simulink model "controller_imp"  (R2024b)
settings: Solver=FixedStepDiscrete  StartTime=0.0  StopTime=1000  FixedStep=1/10  RelTol=1e-3  EnableMultiTasking=on
undefined symbols (not defined in the file): MAX_RDB_ENGAGE_SPEED, MAX_TORQUE, MAX_TORQUE_REVERSE, TransmissionState
libraries: arduinolib x18
settings Model: ExtModeTrigDuration=2  Creator=DAUIN-Win10  LastModifiedBy=feder
settings SolverCC: AutoInsertRateTranBlk=on
settings OptimizationCC: EnhancedBackFolding=on  PassReuseOutputArgsAs=Individual arguments  ZeroExternalMemoryAtStartup=off  ZeroInternalMemoryAtStartup=off  MaxStackSize=64  OptimizeBlockOrder=speed  DifferentSizesBufferReuse=on  OptimizationCustomize=off  EfficientTunableParamExpr=on
settings DebuggingCC: ParameterTunabilityLossMsg=error  UnconnectedInputMsg=warning  UnconnectedOutputMsg=warning  UnconnectedLineMsg=warning
settings HardwareCC: ProdBitPerInt=16  ProdBitPerPointer=16  ProdBitPerSizeT=16  ProdBitPerPtrDiffT=16  ProdLargestAtomicFloat=None  ProdWordSize=8  ProdHWDeviceType=Atmel->AVR
settings ModelReferenceCC: EnableRefExpFcnMdlSchedulingChecks=on
settings SFSimCC: MATLABDynamicMemAlloc=off
settings RTWCC: Description=Embedded Coder  SystemTargetFile=ert.tlc  HardwareBoard=Arduino Uno  TemplateMakefile=ert_default_tmf  Toolchain=Arduino AVR  BuildConfiguration=Faster Runs  GPUComputeCapability=3.5  DLArmComputeVersion=19.05
settings CodeAppCC: ForceParamTrailComments=on  IgnoreCustomStorageClasses=off  OperatorAnnotations=on  SimulinkDataObjDesc=on  SFDataObjDesc=on  InsertBlockDesc=on
settings ERTTargetCC: SupportVariableSizeSignals=on  ExtModeTransport=3  ExtModeStaticAlloc=on  ExtModeAutomaticAllocSize=off  ExtModeStaticAllocSize=250  ExtModeMexFile=ext_xcp  ExtModeIntrfLevel=Level2 - Open  InlinedParameterPlacement=Hierarchical

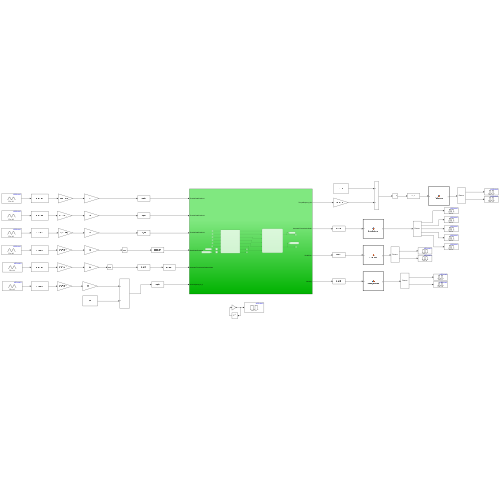
[thumbnail: Simulink's stored preview of the top-level diagram]
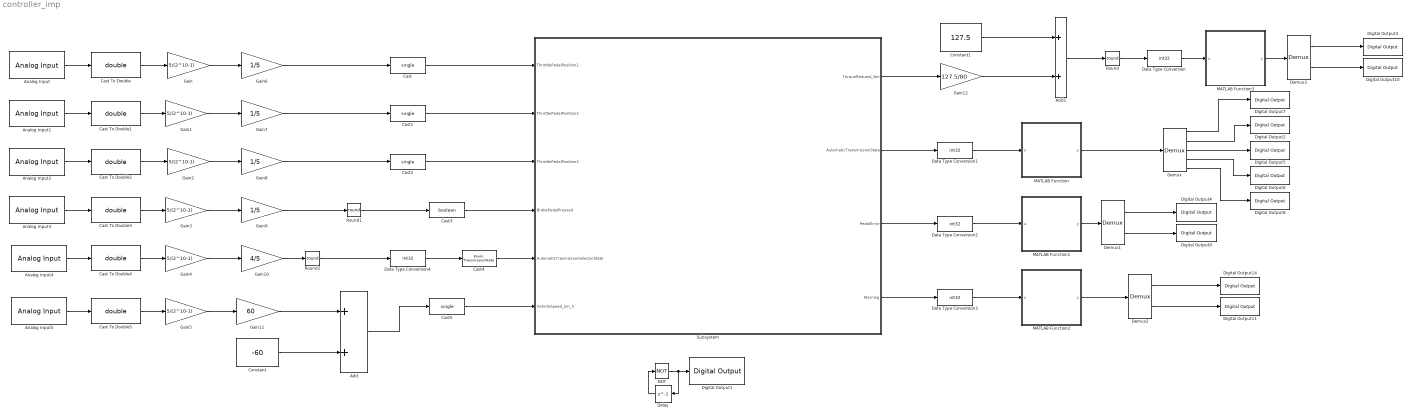
== system controller_imp ==
  Add : Sum
  Add1 : Sum
  Analog Input : arduinolib/Analog Input  pinNumber=1  ReadResultsOnly=off  ConversionTriggerSource=Software  ExternalTriggerType=uint32( 0 )  OutputDataType=uint16  EnableConversionCompleteNotify=off  EnableOuputStatus=off  SampleTime=-1  blockPlatform=arduino
      settings: SourceProductName=Common
  Analog Input1 : arduinolib/Analog Input  pinNumber=2  ReadResultsOnly=off  ConversionTriggerSource=Software  ExternalTriggerType=uint32( 0 )  OutputDataType=uint16  EnableConversionCompleteNotify=off  EnableOuputStatus=off  SampleTime=-1  blockPlatform=arduino
      settings: SourceProductName=Common
  Analog Input2 : arduinolib/Analog Input  pinNumber=3  ReadResultsOnly=off  ConversionTriggerSource=Software  ExternalTriggerType=uint32( 0 )  OutputDataType=uint16  EnableConversionCompleteNotify=off  EnableOuputStatus=off  SampleTime=-1  blockPlatform=arduino
      settings: SourceProductName=Common
  Analog Input3 : arduinolib/Analog Input  pinNumber=0  ReadResultsOnly=off  ConversionTriggerSource=Software  ExternalTriggerType=uint32( 0 )  OutputDataType=uint16  EnableConversionCompleteNotify=off  EnableOuputStatus=off  SampleTime=-1  blockPlatform=arduino
      settings: SourceProductName=Common
  Analog Input4 : arduinolib/Analog Input  pinNumber=4  ReadResultsOnly=off  ConversionTriggerSource=Software  ExternalTriggerType=uint32( 0 )  OutputDataType=uint16  EnableConversionCompleteNotify=off  EnableOuputStatus=off  SampleTime=-1  blockPlatform=arduino
      settings: SourceProductName=Common
  Analog Input5 : arduinolib/Analog Input  pinNumber=5  ReadResultsOnly=off  ConversionTriggerSource=Software  ExternalTriggerType=uint32( 0 )  OutputDataType=uint16  EnableConversionCompleteNotify=off  EnableOuputStatus=off  SampleTime=-1  blockPlatform=arduino
      settings: SourceProductName=Common
  Cast{,1..2,5} (4 alike) : DataTypeConversion  OutDataTypeStr=single  SaturateOnIntegerOverflow=off  RndMeth=Floor
  Cast To Double{,1..5} (6 alike) : DataTypeConversion  OutDataTypeStr=double  SaturateOnIntegerOverflow=off  RndMeth=Floor
  Cast3 : DataTypeConversion  OutDataTypeStr=boolean  SaturateOnIntegerOverflow=off  RndMeth=Floor
  Cast4 : DataTypeConversion  OutDataTypeStr=Enum: TransmissionState  SaturateOnIntegerOverflow=off  RndMeth=Floor
  Constant : Constant  Value=-60
  Constant1 : Constant  Value=127.5  OutDataTypeStr=Inherit: Inherit via back propagation
  Data Type Conversion{,1..4} (5 alike) : DataTypeConversion  OutDataTypeStr=int32  SaturateOnIntegerOverflow=off  RndMeth=Floor
  Delay : Delay  DelayLength=1  InputProcessing=Columns as channels (frame based)
  Demux : Demux  Outputs=5
      settings: DisplayOption=none
  Demux1 : Demux  Outputs=2
      settings: DisplayOption=none
  Demux2 : Demux  Outputs=2
      settings: DisplayOption=none
  Demux3 : Demux  Outputs=2
      settings: DisplayOption=none
  Digital Output1 : arduinolib/Digital Output  pinNumber=13  Direction=output  blockPlatform=arduino
      settings: SourceProductName=Common
  Digital Output10 : arduinolib/Digital Output  pinNumber=12  Direction=output  blockPlatform=arduino
      settings: SourceProductName=Common
  Digital Output11 : arduinolib/Digital Output  pinNumber=10  Direction=output  blockPlatform=arduino
      settings: SourceProductName=Common
  Digital Output14 : arduinolib/Digital Output  pinNumber=9  Direction=output  blockPlatform=arduino
      settings: SourceProductName=Common
  Digital Output2 : arduinolib/Digital Output  pinNumber=3  Direction=output  blockPlatform=arduino
      settings: SourceProductName=Common
  Digital Output3 : arduinolib/Digital Output  pinNumber=11  Direction=output  blockPlatform=arduino
      settings: SourceProductName=Common
  Digital Output4 : arduinolib/Digital Output  pinNumber=7  Direction=output  blockPlatform=arduino
      settings: SourceProductName=Common
  Digital Output5 : arduinolib/Digital Output  pinNumber=4  Direction=output  blockPlatform=arduino
      settings: SourceProductName=Common
  Digital Output6 : arduinolib/Digital Output  pinNumber=5  Direction=output  blockPlatform=arduino
      settings: SourceProductName=Common
  Digital Output7 : arduinolib/Digital Output  pinNumber=2  Direction=output  blockPlatform=arduino
      settings: SourceProductName=Common
  Digital Output8 : arduinolib/Digital Output  pinNumber=6  Direction=output  blockPlatform=arduino
      settings: SourceProductName=Common
  Digital Output9 : arduinolib/Digital Output  pinNumber=8  Direction=output  blockPlatform=arduino
      settings: SourceProductName=Common
  Gain{,1..5} (6 alike) : Gain  Gain=5/(2^10-1)
  Gain10 : Gain  Gain=4/5
  Gain11 : Gain  Gain=60
  Gain12 : Gain  Gain=127.5/80
  Gain{6..9} (4 alike) : Gain  Gain=1/5
  MATLAB Function : MATLAB Function  TreatAsAtomicUnit=on
  MATLAB Function1 : MATLAB Function  TreatAsAtomicUnit=on
  MATLAB Function2 : MATLAB Function  TreatAsAtomicUnit=on
  MATLAB Function3 : MATLAB Function  TreatAsAtomicUnit=on
  NOT : Logic  Operator=NOT  IconShape=distinctive  AllPortsSameDT=off  OutDataTypeStr=boolean
  Round : Rounding  Operator=round
  Round1 : Rounding  Operator=round
  Round2 : Rounding  Operator=round
  Subsystem : Subsystem
  wires:
  Subsystem/3(PedalError) -> Data Type Conversion2/1
  Cast To Double1/1 -> Gain1/1
  Add1/1 -> Round/1
  NOT/1 -> Delay/1, Digital Output1/1
  Gain12/1 -> Add1/2
  Cast5/1 -> Subsystem/6(VehicleSpeed_km_h)
  MATLAB Function1/1(y) -> Demux1/1
  Subsystem/4(Warning) -> Data Type Conversion3/1
  Analog Input3/1 -> Cast To Double3/1
  Round/1 -> Data Type Conversion/1
  Gain5/1 -> Gain11/1
  Cast To Double5/1 -> Gain5/1
  Cast To Double/1 -> Gain/1
  Analog Input4/1 -> Cast To Double4/1
  MATLAB Function2/1(y) -> Demux2/1
  Gain/1 -> Gain6/1
  Round2/1 -> Data Type Conversion4/1
  Analog Input/1 -> Cast To Double/1
  Gain7/1 -> Cast1/1
  Analog Input5/1 -> Cast To Double5/1
  Cast2/1 -> Subsystem/3(ThrottlePedalPosition3)
  Round1/1 -> Cast3/1
  Demux/2 -> Digital Output2/1
  Add/1 -> Cast5/1
  Gain10/1 -> Round2/1
  Cast To Double3/1 -> Gain3/1
  Gain8/1 -> Cast2/1
  Gain4/1 -> Gain10/1
  Demux1/1 -> Digital Output4/1
  Cast4/1 -> Subsystem/5(AutomaticTrasmissionSelectorState)
  Demux/1 -> Digital Output7/1
  Demux/3 -> Digital Output5/1
  Gain1/1 -> Gain7/1
  Gain2/1 -> Gain8/1
  Constant1/1 -> Add1/1
  Analog Input2/1 -> Cast To Double2/1
  Data Type Conversion4/1 -> Cast4/1
  Cast To Double4/1 -> Gain4/1
  Subsystem/2(AutomaticTransmissionState) -> Data Type Conversion1/1
  Demux/5 -> Digital Output8/1
  Demux1/2 -> Digital Output9/1
  Cast1/1 -> Subsystem/2(ThrottlePedalPosition2)
  Cast3/1 -> Subsystem/4(BrakePedalPressed)
  Gain9/1 -> Round1/1
  MATLAB Function/1(y) -> Demux/1
  Data Type Conversion3/1 -> MATLAB Function2/1(u)
  Constant/1 -> Add/2
  Analog Input1/1 -> Cast To Double1/1
  Gain6/1 -> Cast/1
  Cast To Double2/1 -> Gain2/1
  Data Type Conversion1/1 -> MATLAB Function/1(u)
  Gain3/1 -> Gain9/1
  Subsystem/1(TorqueRequest_Nm) -> Gain12/1
  Data Type Conversion2/1 -> MATLAB Function1/1(u)
  Gain11/1 -> Add/1
  Demux2/2 -> Digital Output11/1
  Delay/1 -> NOT/1
  Cast/1 -> Subsystem/1(ThrottlePedalPosition1)
  Demux/4 -> Digital Output6/1
  Demux2/1 -> Digital Output14/1
  Data Type Conversion/1 -> MATLAB Function3/1(u)
  Demux3/2 -> Digital Output10/1
  Demux3/1 -> Digital Output3/1
  MATLAB Function3/1(y) -> Demux3/1

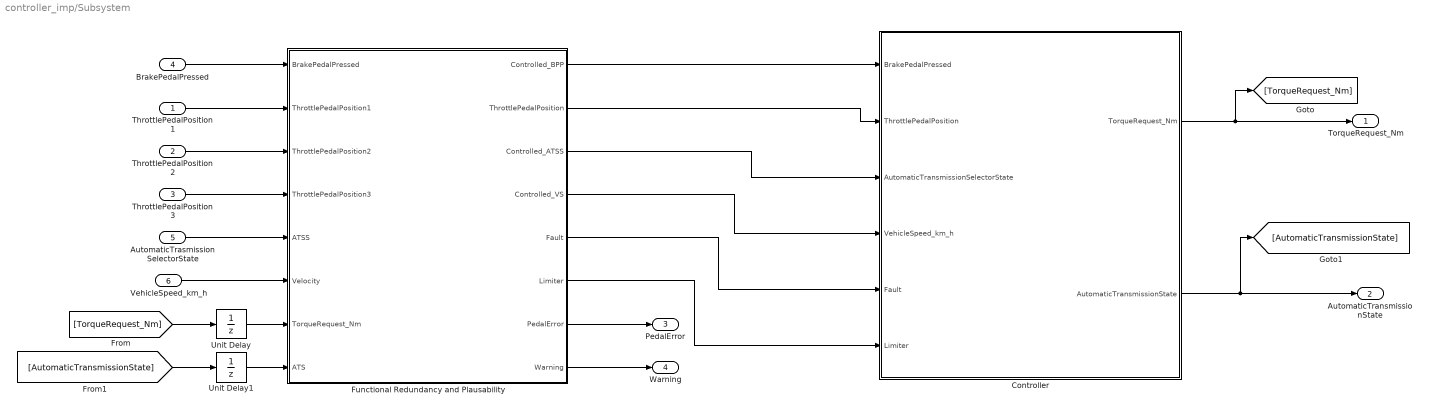
== system controller_imp/Subsystem ==
  ThrottlePedalPosition1 : Inport  OutDataTypeStr=single
  ThrottlePedalPosition2 : Inport  Port=2  OutDataTypeStr=single
  ThrottlePedalPosition3 : Inport  Port=3  OutDataTypeStr=single
  BrakePedalPressed : Inport  Port=4  OutDataTypeStr=boolean
  AutomaticTrasmissionSelectorState : Inport  Port=5  OutDataTypeStr=Enum: TransmissionState
  VehicleSpeed_km_h : Inport  Port=6  OutDataTypeStr=single  Unit=km/h
  Controller : Stateflow chart  TreatAsAtomicUnit=on
      settings: PortSchema="{\"entries\":[{\"content\":{\"sides\":[{\"content\":{\"connectorIds\":[\"In1\",\"In2\",\"In3\",\"In5\",\"In4\",\"In6\"]},\"type\":\"ConnectorPlacement.EquallySpacedRectSide\",\"uuid\":\"8299657d-0502-40c6-b0a0-94f373f4d980\"},{\"content\":{\"connectorIds\":[\"Out1\",\"Out2\"],\"side\":\"RIGHT\"},\"type\":\"ConnectorPlacement.EquallySpacedRectSide\",\"uuid\":\"5efbfe3b-c679-4c7a-ba60-d200927433b8\"},{\"content\":{\"side\":\"TOP\"},\"type\":\"ConnectorPlacement.EquallySpacedRectSide\",\"uuid\":\"8eb3a2db-d3ff-40e0-8198-21b1625c1f86\"}]},\"type\":\"ConnectorPlacement.EquallySpacedConnector\",\"uuid\":\"73ac7723-3127-41a8-b70c-f20bcd517ff0\"}],\"packageUris\":[\"http://schema.mathworks.com/mf0/Connector/R2020b\"],\"version\":\"1.0\"}"
  Functional Redundancy and Plausability : Subsystem
  Unit Delay : UnitDelay  SampleTime=-1  HasFrameUpgradeWarning=on
  Unit Delay1 : UnitDelay  InitialCondition=TransmissionState.Park  SampleTime=-1  HasFrameUpgradeWarning=on
  TorqueRequest_Nm : Outport  OutDataTypeStr=single  Unit=N*m
  AutomaticTransmissionState : Outport  Port=2  OutDataTypeStr=Enum: TransmissionState
  PedalError : Outport  Port=3  OutDataTypeStr=single
  Warning : Outport  Port=4  OutDataTypeStr=Enum: WarningType
  wires:
  Functional Redundancy and Plausability/4(Controlled_VS) -> Controller/5(VehicleSpeed_km_h)
  Functional Redundancy and Plausability/7(PedalError) -> PedalError/1
  Functional Redundancy and Plausability/2(ThrottlePedalPosition) -> Controller/2(ThrottlePedalPosition)
  Functional Redundancy and Plausability/8(Warning) -> Warning/1
  ThrottlePedalPosition3/1 -> Functional Redundancy and Plausability/4(ThrottlePedalPosition3)
  ThrottlePedalPosition2/1 -> Functional Redundancy and Plausability/3(ThrottlePedalPosition2)
  Controller/2(AutomaticTransmissionState) -> AutomaticTransmissionState/1, [AutomaticTransmissionState]
  Unit Delay1/1 -> Functional Redundancy and Plausability/8(ATS)
  ThrottlePedalPosition1/1 -> Functional Redundancy and Plausability/2(ThrottlePedalPosition1)
  Functional Redundancy and Plausability/1(Controlled_BPP) -> Controller/1(BrakePedalPressed)
  [TorqueRequest_Nm] -> Unit Delay/1
  Functional Redundancy and Plausability/5(Fault) -> Controller/4(Fault)
  Functional Redundancy and Plausability/3(Controlled_ATSS) -> Controller/3(AutomaticTransmissionSelectorState)
  Controller/1(TorqueRequest_Nm) -> TorqueRequest_Nm/1, [TorqueRequest_Nm]
  Unit Delay/1 -> Functional Redundancy and Plausability/7(TorqueRequest_Nm)
  BrakePedalPressed/1 -> Functional Redundancy and Plausability/1(BrakePedalPressed)
  [AutomaticTransmissionState] -> Unit Delay1/1
  Functional Redundancy and Plausability/6(Limiter) -> Controller/6(Limiter)
  VehicleSpeed_km_h/1 -> Functional Redundancy and Plausability/6(Velocity)
  AutomaticTrasmissionSelectorState/1 -> Functional Redundancy and Plausability/5(ATSS)

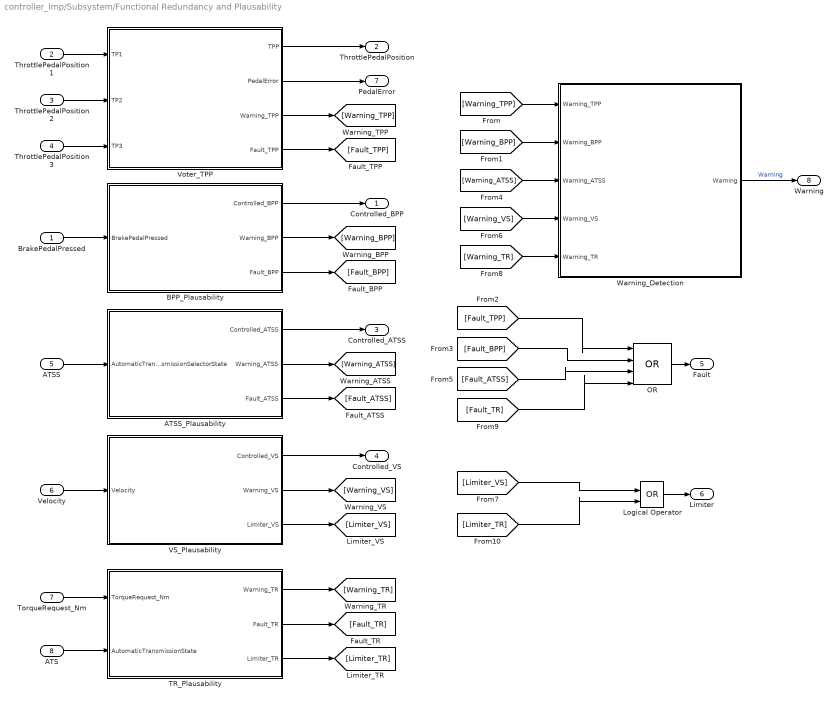
== system controller_imp/Subsystem/Functional Redundancy and Plausability ==
  BrakePedalPressed : Inport
  ThrottlePedalPosition1 : Inport  Port=2
  ThrottlePedalPosition2 : Inport  Port=3
  ThrottlePedalPosition3 : Inport  Port=4
  ATSS : Inport  Port=5  OutDataTypeStr=Enum: TransmissionState
  Velocity : Inport  Port=6  OutDataTypeStr=single
  TorqueRequest_Nm : Inport  Port=7  OutDataTypeStr=single
  ATS : Inport  Port=8  OutDataTypeStr=Enum: TransmissionState
  ATSS_Plausability : MATLAB Function  TreatAsAtomicUnit=on
  BPP_Plausability : MATLAB Function  TreatAsAtomicUnit=on
  Logical Operator : Logic  Operator=OR  IconShape=distinctive  AllPortsSameDT=off  OutDataTypeStr=boolean
  OR : Logic  Operator=OR  Inputs=4  IconShape=distinctive  AllPortsSameDT=off  OutDataTypeStr=boolean
  TR_Plausability : MATLAB Function  TreatAsAtomicUnit=on
  VS_Plausability : MATLAB Function  TreatAsAtomicUnit=on
  Voter_TPP : MATLAB Function  TreatAsAtomicUnit=on
  Warning_Detection : MATLAB Function  TreatAsAtomicUnit=on
  Controlled_BPP : Outport  OutDataTypeStr=boolean
  ThrottlePedalPosition : Outport  Port=2  OutMin=[0]  OutMax=[1]
  Controlled_ATSS : Outport  Port=3  OutDataTypeStr=Enum: TransmissionState
  Controlled_VS : Outport  Port=4  OutDataTypeStr=single
  Fault : Outport  Port=5  OutDataTypeStr=boolean
  Limiter : Outport  Port=6  OutDataTypeStr=boolean
  PedalError : Outport  Port=7  OutDataTypeStr=single
  Warning : Outport  Port=8  OutDataTypeStr=Enum: WarningType
  wires:
  ThrottlePedalPosition1/1 -> Voter_TPP/1(TP1)
  ThrottlePedalPosition2/1 -> Voter_TPP/2(TP2)
  ThrottlePedalPosition3/1 -> Voter_TPP/3(TP3)
  Voter_TPP/1(TPP) -> ThrottlePedalPosition/1
  Voter_TPP/2(PedalError) -> PedalError/1
  BrakePedalPressed/1 -> BPP_Plausability/1(BrakePedalPressed)
  BPP_Plausability/1(Controlled_BPP) -> Controlled_BPP/1
  Velocity/1 -> VS_Plausability/1(Velocity)
  VS_Plausability/1(Controlled_VS) -> Controlled_VS/1
  ATSS/1 -> ATSS_Plausability/1(AutomaticTransmissionSelectorState)
  ATSS_Plausability/1(Controlled_ATSS) -> Controlled_ATSS/1
  TorqueRequest_Nm/1 -> TR_Plausability/1(TorqueRequest_Nm)
  ATS/1 -> TR_Plausability/2(AutomaticTransmissionState)
  OR/1 -> Fault/1
  Voter_TPP/3(Warning_TPP) -> [Warning_TPP]
  BPP_Plausability/2(Warning_BPP) -> [Warning_BPP]
  ATSS_Plausability/2(Warning_ATSS) -> [Warning_ATSS]
  VS_Plausability/2(Warning_VS) -> [Warning_VS]
  TR_Plausability/1(Warning_TR) -> [Warning_TR]
  Voter_TPP/4(Fault_TPP) -> [Fault_TPP]
  BPP_Plausability/3(Fault_BPP) -> [Fault_BPP]
  ATSS_Plausability/3(Fault_ATSS) -> [Fault_ATSS]
  TR_Plausability/2(Fault_TR) -> [Fault_TR]
  VS_Plausability/3(Limiter_VS) -> [Limiter_VS]
  TR_Plausability/3(Limiter_TR) -> [Limiter_TR]
  [Warning_TPP] -> Warning_Detection/1(Warning_TPP)
  [Warning_ATSS] -> Warning_Detection/3(Warning_ATSS)
  [Warning_VS] -> Warning_Detection/4(Warning_VS)
  [Warning_TR] -> Warning_Detection/5(Warning_TR)
  Warning_Detection/1(Warning) -> Warning/1  "Warning"
  [Fault_TPP] -> OR/1
  [Fault_TR] -> OR/4
  [Fault_BPP] -> OR/2
  [Fault_ATSS] -> OR/3
  [Limiter_VS] -> Logical Operator/1
  [Limiter_TR] -> Logical Operator/2
  Logical Operator/1 -> Limiter/1
  [Warning_BPP] -> Warning_Detection/2(Warning_BPP)

== matlab function controller_imp/Subsystem/Functional Redundancy and Plausability/VS_Plausability ==
  data: Velocity input single; Controlled_VS output single; Warning_VS output Enum: WarningType; Limiter_VS output boolean
function [Controlled_VS,Warning_VS,Limiter_VS] = VS_Plausability(Velocity)

Controlled_VS = single(Velocity);
Warning_VS =  WarningType(0);
Limiter_VS = boolean(0);

if (Velocity > 240 || Velocity < -60)

    Warning_VS =  WarningType(1);
    Limiter_VS = boolean(1);

end

== matlab function controller_imp/Subsystem/Functional Redundancy and Plausability/BPP_Plausability ==
  data: BrakePedalPressed input; Controlled_BPP output; Warning_BPP output Enum: WarningType; Fault_BPP output boolean
function [Controlled_BPP,Warning_BPP,Fault_BPP] = BPP_Plausability(BrakePedalPressed)

Warning_BPP = WarningType(0);
Fault_BPP = boolean(0);
Controlled_BPP = boolean(0);

if (BrakePedalPressed == 0 || BrakePedalPressed == 1) 

    Controlled_BPP = boolean(BrakePedalPressed);
        
else

    Warning_BPP = WarningType(2);
    Fault_BPP = boolean(1);

end

== stateflow chart controller_imp/Subsystem/Controller ==
  state Park
    entry:
    AutomaticTransmissionState = TransmissionState.Park;
    during:
    TorqueRequest_Nm = 0;
  state Reverse
    entry:
    AutomaticTransmissionState = TransmissionState.Reverse;
    state BackwardAcceleration
      during:
      TorqueRequest_Nm = -MAX_TORQUE_REVERSE*ThrottlePedalPosition;
    state BackwardRestart
      during:
      TorqueRequest_Nm = -MAX_TORQUE_REVERSE/20;
    state Limiter
      during:
      TorqueRequest_Nm = 0;
    state Stop
      during:
      TorqueRequest_Nm = 0;
    (default) -> BackwardAcceleration
    BackwardRestart -> BackwardAcceleration : [BrakePedalPressed == 0 && ThrottlePedalPosition > 0]
    BackwardAcceleration -> Reverse.Stop [order 1] : [BrakePedalPressed == 1]
    Reverse.Stop -> BackwardAcceleration [order 2] : [BrakePedalPressed == 0]
    (junction 219) -> BackwardAcceleration
    BackwardAcceleration -> (junction 215) [order 2]
    (junction 77) -> BackwardRestart
    (junction 215) -> Reverse.Limiter : [Limiter == 1]
    Reverse.Limiter -> (junction 219) : [Limiter == 0]
    Reverse.Stop -> (junction 77) [order 1] : [BrakePedalPressed == 0 && abs(VehicleSpeed_km_h) <= MAX_RDB_ENGAGE_SPEED]
  state Brake
    entry:
    AutomaticTransmissionState = TransmissionState.Brake;
    state Acceleration
      during:
      TorqueRequest_Nm = MAX_TORQUE*3/2*(ThrottlePedalPosition-1/3);
    state Restart
      during:
      TorqueRequest_Nm = MAX_TORQUE/20;
    state EmergencyStop
      during:
      TorqueRequest_Nm = 0;
    state Stop
      during:
      TorqueRequest_Nm = 0;
    state RegenarativeBraking
      during:
      TorqueRequest_Nm = -MAX_TORQUE*(1-3*ThrottlePedalPosition);
    (default) -> Brake.Acceleration
    Brake.Restart -> Brake.Acceleration [order 2] : [VehicleSpeed_km_h > MAX_RDB_ENGAGE_SPEED]
    Brake.Acceleration -> (junction 123) [order 2] : [BrakePedalPressed == 1 || Limiter == 1]
    (junction 123) -> EmergencyStop
    Brake.Acceleration -> RegenarativeBraking [order 1] : [ThrottlePedalPosition <= 1/3]
    RegenarativeBraking -> Brake.Acceleration [order 1] : [ThrottlePedalPosition > 1/3]
    Brake.Restart -> Brake.Stop [order 1] : [ThrottlePedalPosition <= 1/3 || BrakePedalPressed ==1]
    Brake.Stop -> Brake.Restart [order 1] : [ThrottlePedalPosition > 1/3]
    EmergencyStop -> (junction 127) : [BrakePedalPressed == 0 && Limiter == 0]
    (junction 127) -> RegenarativeBraking
    (junction 134) -> EmergencyStop
    (junction 190) -> EmergencyStop
    RegenarativeBraking -> (junction 134) [order 3] : [BrakePedalPressed == 1]
    Brake.Stop -> (junction 190) [order 2] : [BrakePedalPressed == 1]
    RegenarativeBraking -> Brake.Stop [order 2] : [VehicleSpeed_km_h <= MAX_RDB_ENGAGE_SPEED]
  state Drive
    entry:
    AutomaticTransmissionState = TransmissionState.Drive;
    state Acceleration
      during:
      TorqueRequest_Nm = MAX_TORQUE*ThrottlePedalPosition;
    state Restart
      during:
      TorqueRequest_Nm = MAX_TORQUE/20;
    state Limiter
      during:
      TorqueRequest_Nm = 0;
    state Stop
      during:
      TorqueRequest_Nm = 0;
    (default) -> Drive.Acceleration
    Drive.Restart -> Drive.Acceleration : [BrakePedalPressed == 0 && ThrottlePedalPosition > 0]
    Drive.Acceleration -> Drive.Stop [order 1] : [BrakePedalPressed == 1]
    Drive.Stop -> Drive.Acceleration [order 2] : [BrakePedalPressed == 0]
    (junction 211) -> Drive.Acceleration
    Drive.Acceleration -> (junction 208) [order 2]
    (junction 62) -> Drive.Restart
    (junction 208) -> Drive.Limiter : [Limiter == 1]
    Drive.Limiter -> (junction 211) : [Limiter == 0]
    Drive.Stop -> (junction 62) [order 1] : [BrakePedalPressed == 0 && VehicleSpeed_km_h <= MAX_RDB_ENGAGE_SPEED]
  state Neutral
    entry:
    AutomaticTransmissionState = TransmissionState.Neutral;
    during:
    TorqueRequest_Nm = 0;
  (default) -> Park
  Neutral -> Park [order 3] : [abs(VehicleSpeed_km_h) < 5 && BrakePedalPressed == 1 && AutomaticTransmissionSelectorState == 0 && Fault == 0]
  Park -> Neutral : [BrakePedalPressed == 1 && AutomaticTransmissionSelectorState ~= 0 || Fault == 1]
  Brake -> Drive : [AutomaticTransmissionSelectorState ~= 4 || Fault == 1]
  Drive -> Neutral [order 1] : [AutomaticTransmissionSelectorState == 0 || AutomaticTransmissionSelectorState == 1 || AutomaticTransmissionSelectorState == 2 || Fault == 1]
  Neutral -> Reverse [order 2] : [VehicleSpeed_km_h < 5 && BrakePedalPressed == 1 && AutomaticTransmissionSelectorState == 1 && Fault == 0]
  Reverse -> Neutral : [AutomaticTransmissionSelectorState ~= 1 || Fault == 1]
  Neutral -> Drive [order 1] : [VehicleSpeed_km_h > -5 && BrakePedalPressed == 1 && (AutomaticTransmissionSelectorState == 4|| AutomaticTransmissionSelectorState == 3) && Fault == 0 ]
  Drive -> Brake [order 2] : [ThrottlePedalPosition > 1/3 && AutomaticTransmissionSelectorState == 4 && Fault == 0]
  data: BrakePedalPressed input boolean; ThrottlePedalPosition input single; AutomaticTransmissionSelectorState input Enum: TransmissionState; Fault input boolean; MAX_TORQUE parameter single; MAX_RDB_ENGAGE_SPEED parameter single; TorqueRequest_Nm output single; AutomaticTransmissionState output Enum: TransmissionState; VehicleSpeed_km_h input single; MAX_TORQUE_REVERSE parameter single; Limiter input boolean

== matlab function controller_imp/Subsystem/Functional Redundancy and Plausability/ATSS_Plausability ==
  data: AutomaticTransmissionSelectorState input; Controlled_ATSS output Enum: TransmissionState; Warning_ATSS output Enum: WarningType; Fault_ATSS output
function [Controlled_ATSS,Warning_ATSS,Fault_ATSS] = ATSS_Plausability(AutomaticTransmissionSelectorState)

Controlled_ATSS = TransmissionState(2);
Warning_ATSS = WarningType(0);
Fault_ATSS = boolean(0);

ValidModes = [0 1 2 3 4];

if any(AutomaticTransmissionSelectorState == ValidModes)

    Controlled_ATSS = TransmissionState(AutomaticTransmissionSelectorState);
    
else

    Warning_ATSS = WarningType(2);
    Fault_ATSS = boolean(1);

end

== matlab function controller_imp/Subsystem/Functional Redundancy and Plausability/Voter_TPP ==
  data: TPP output; PedalError output; TP1 input; Warning_TPP output Enum: WarningType; TP2 input; TP3 input; Fault_TPP output
function [TPP,PedalError,Warning_TPP,Fault_TPP] = Voter_TPP(TP1,TP2,TP3)

% Initialization of the output
TPP = single(0);
Warning_TPP = WarningType(0);
PedalError = single(0);
Fault_TPP = boolean(0);
comp = 0.02;

% Comparison between the signals
Diff_1_2 = abs(TP1-TP2);
Diff_1_3 = abs(TP1-TP3);
Diff_2_3 = abs(TP2-TP3);

if (Diff_1_2 <= comp && Diff_1_3 <= comp)

    TPP = (TP1 + TP2 + TP3)/3;
    
elseif Diff_1_2 <= comp

    TPP = (TP1 + TP2)/2;
    Warning_TPP = WarningType(1);
    PedalError = single(3);

elseif Diff_1_3 <= comp

    TPP = (TP1 + TP3)/2;
    Warning_TPP = WarningType(1);
    PedalError = single(2);

elseif Diff_2_3 <= comp

    TPP = (TP2 + TP3)/2;
    Warning_TPP = WarningType(1);
    PedalError = single(1);

else
    
    TPP = single(0);
    Warning_TPP = WarningType(2);
    Fault_TPP = boolean(1);    
    PedalError = single(4);

end

== matlab function controller_imp/Subsystem/Functional Redundancy and Plausability/TR_Plausability ==
  data: Warning_TR output Enum: WarningType; TorqueRequest_Nm input single; Fault_TR output boolean; AutomaticTransmissionState input; Limiter_TR output boolean
function [Warning_TR,Fault_TR,Limiter_TR] = TR_Plausability(TorqueRequest_Nm,AutomaticTransmissionState)

Warning_TR = WarningType(0);
Fault_TR = boolean(0);
Limiter_TR = boolean(0);

PositiveMode = [TransmissionState.Drive, TransmissionState.Brake];
NegativeMode = [TransmissionState.Reverse, TransmissionState.Brake];

if ((TorqueRequest_Nm == 0 ) ...
        || (TorqueRequest_Nm > 0 && any(AutomaticTransmissionState == PositiveMode)) ...
        || (TorqueRequest_Nm < 0  && any(AutomaticTransmissionState == NegativeMode)))
    
    if (TorqueRequest_Nm > 80 || TorqueRequest_Nm < -80 )
        
        Warning_TR =  WarningType(1);
        Limiter_TR = boolean(1);
        
    end

else

    Warning_TR =  WarningType(2);
    Fault_TR = boolean(1); 

end

== matlab function controller_imp/Subsystem/Functional Redundancy and Plausability/Warning_Detection ==
  data: Warning_TPP input Enum: WarningType; Warning output Enum: WarningType; Warning_BPP input Enum: WarningType; Warning_ATSS input Enum: WarningType; Warning_VS input Enum: WarningType; Warning_TR input Enum: WarningType
function Warning = Warning_Detection(Warning_TPP,Warning_BPP,Warning_ATSS,Warning_VS,Warning_TR)

Warning =  WarningType(0);

Warning_set = [Warning_TPP,Warning_BPP,Warning_ATSS,Warning_VS,Warning_TR];

if any(Warning_set ==  WarningType(1))

    Warning =  WarningType(1);

     if any(Warning_set == WarningType(2))
    
        Warning = WarningType(2);
    
     end

elseif any(Warning_set == WarningType(2))

    Warning = WarningType(2);

end

== matlab function controller_imp/MATLAB Function ==
  data: u input; y output
function y = StateSelector(u)

y = false(1,5);

if u >= 0 && u <= 4
    
    y(u+1) = true;

end

== matlab function controller_imp/MATLAB Function1 ==
  data: u input; y output
function y = PESelector(u)

y = false(1,2);

if u >= 1 && u <= 3
    
    y(1) = true;

elseif u == 4

     y(2) = true;

end

== matlab function controller_imp/MATLAB Function2 ==
  data: u input; y output
function y = WarningSelector(u)

y = false(1,2);

if u > 0

    y = [false true];

    if u == 1

        y = [true true];
    
    end

end

== matlab function controller_imp/MATLAB Function3 ==
  data: u input; y output
function y = TRSelector(u)

y = false(1,2);

if u >= 128
    
    y(1) = true;

elseif u < 128

    y(2) = true;

end
